simulink model "sf_basic"  (R2015b)
settings: Solver=FixedStepDiscrete  SolverMode=SingleTasking  StartTime=0.0  StopTime=1  RelTol=1e-3
settings Model: Creator=at-mt  LastModifiedBy=amatsumo
settings DataIOCC: SaveFormat=Array  SignalLoggingSaveFormat=ModelDataLogs  SaveOutput=off  SignalLogging=off  SaveTime=off
settings OptimizationCC: BlockReduction=off  ConditionallyExecuteInputs=off  DefaultParameterBehavior=Inlined  ExpressionDepthLimit=2147483647
settings DebuggingCC: AlgebraicLoopMsg=error  UnderspecifiedInitializationDetection=Classic  MergeDetectMultiDrivingBlocksExec=none  SolverPrmCheckMsg=warning  SingleTaskRateTransMsg=error  FcnCallInpInsideContextMsg=UseLocalSettings  StateNameClashWarn=warning
settings HardwareCC: ProdBitPerPointer=32  ProdLargestAtomicFloat=None  ProdIntDivRoundTo=Undefined  ProdEndianess=Unspecified  ProdWordSize=32  ProdHWDeviceType=ASIC/FPGA->ASIC/FPGA  TargetBitPerPointer=64  TargetLongLongMode=on  TargetIntDivRoundTo=Zero  TargetEndianess=LittleEndian  TargetWordSize=64  TargetHWDeviceType=MATLAB Host  ProdEqTarget=off
settings GRTTargetCC: GeneratePreprocessorConditionals=Disable all  CombineOutputUpdateFcns=off  GRTInterface=on
settings ConfigComp: CovModelRefEnable=Off  CovSFcnEnable=off

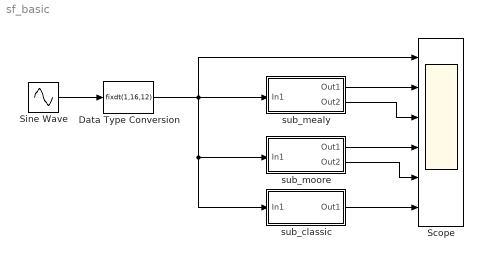
== system sf_basic ==
  Data Type Conversion : DataTypeConversion  OutDataTypeStr=fixdt(1,16,12)
  Scope : Scope  NumInputPorts=6
  Sine Wave : Sin  Amplitude=4  Frequency=20  SampleTime=1/100
  sub_classic : Subsystem
  sub_mealy : Subsystem
  sub_moore : Subsystem
  wires:
  Sine Wave/1 -> Data Type Conversion/1
  sub_mealy/1(Out1) -> Scope/2
  Data Type Conversion/1 -> Scope/1, sub_mealy/1(In1), sub_classic/1(In1), sub_moore/1(In1)
  sub_moore/1(Out1) -> Scope/4
  sub_classic/1(Out1) -> Scope/6
  sub_mealy/2(Out2) -> Scope/3
  sub_moore/2(Out2) -> Scope/5

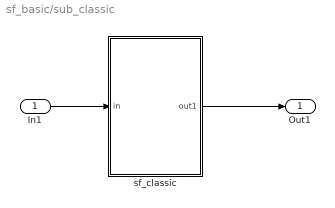
== system sf_basic/sub_classic ==
  In1 : Inport
  sf_classic : Stateflow chart  TreatAsAtomicUnit=on
  Out1 : Outport
  wires:
  In1/1 -> sf_classic/1(in)
  sf_classic/1(out1) -> Out1/1

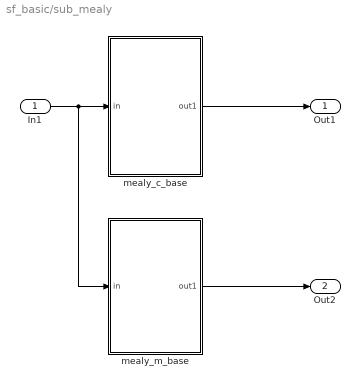
== system sf_basic/sub_mealy ==
  In1 : Inport
  mealy_c_base : Stateflow chart  TreatAsAtomicUnit=on
  mealy_m_base : Stateflow chart  TreatAsAtomicUnit=on
  Out1 : Outport
  Out2 : Outport  Port=2
  wires:
  In1/1 -> mealy_m_base/1(in), mealy_c_base/1(in)
  mealy_c_base/1(out1) -> Out1/1
  mealy_m_base/1(out1) -> Out2/1

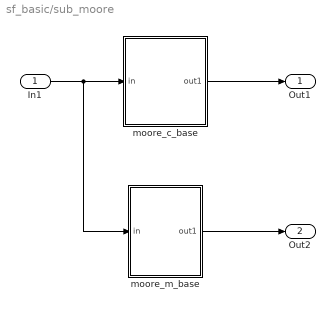
== system sf_basic/sub_moore ==
  In1 : Inport
  moore_c_base : Stateflow chart  TreatAsAtomicUnit=on
  moore_m_base : Stateflow chart  TreatAsAtomicUnit=on
  Out1 : Outport
  Out2 : Outport  Port=2
  wires:
  moore_c_base/1(out1) -> Out1/1
  In1/1 -> moore_m_base/1(in), moore_c_base/1(in)
  moore_m_base/1(out1) -> Out2/1

== stateflow chart sf_basic/sub_mealy/mealy_c_base ==
  settings: updateMethod=DISCRETE  stateMachineType=MEALY_MACHINE  executeAtInitialization=1  initializeOutput=1
  state Init/
  state On1/
  state Off1/
  Init -> Init [order 3] : {out1 = 2;}
  (default) -> Init
  Init -> Off1 [order 2] : [in >= 0]
      | {out1 = 0;}
  On1 -> Init [order 1] : [in >= 0]
      | {out1 = 2;}
  Init -> On1 [order 1] : [in < 0]
      | {out1 = 1;}
  Off1 -> Init [order 1] : [in < 0]
      | {out1 = 2;}
  On1 -> On1 [order 2] : {out1 = 1;}
  Off1 -> Off1 [order 2] : {out1 = 0;}
  data: in input fixdt(1,16,12) size=1; out1 output int16

== stateflow chart sf_basic/sub_moore/moore_m_base ==
  settings: updateMethod=DISCRETE  stateMachineType=MOORE_MACHINE
  state Init/
    out1 = int16(2);
  state On1/
    out1 = int16(1);
  state Off1/
    out1 = int16(0);
  Init -> Init [order 3]
  Init -> Off1 [order 2] : [in >= 0]
  (default) -> Init
  Init -> On1 [order 1] : [in < 0]
  On1 -> Init [order 1] : [in >= 0]
  Off1 -> Init [order 1] : [in < 0]
  On1 -> On1 [order 2]
  Off1 -> Off1 [order 2]
  data: in input fixdt(1,16,12); out1 output int16

== stateflow chart sf_basic/sub_mealy/mealy_m_base ==
  settings: updateMethod=DISCRETE  stateMachineType=MEALY_MACHINE  executeAtInitialization=1  initializeOutput=1
  state Init/
  state On1/
  state Off1/
  Init -> Init [order 3] : {out1 = int16(2);}
  (default) -> Init
  Init -> Off1 [order 2] : [in >= 0]
      | {out1 = int16(0);}
  Init -> On1 [order 1] : [in < 0]
      | {out1 = int16(1);}
  On1 -> Init [order 1] : [in >= 0]
      | {out1 = int16(2);}
  Off1 -> Init [order 1] : [in < 0]
      | {out1 = int16(2);}
  On1 -> On1 [order 2] : {out1 = int16(1);}
  Off1 -> Off1 [order 2] : {out1 = int16(0);}
  data: in input fixdt(1,16,12); out1 output int16

== stateflow chart sf_basic/sub_moore/moore_c_base ==
  settings: updateMethod=DISCRETE  stateMachineType=MOORE_MACHINE  executeAtInitialization=1
  state Init/
    out1 = 2;
  state On1/
    out1 = 1;
  state Off1/
    out1 = 0;
  Init -> Init [order 3]
  Init -> Off1 [order 2] : [in >= 0]
  (default) -> Init
  On1 -> Init [order 1] : [in >= 0]
  Init -> On1 [order 1] : [in < 0]
  Off1 -> Init [order 1] : [in < 0]
  On1 -> On1 [order 2]
  Off1 -> Off1 [order 2]
  data: in input fixdt(1,16,12) size=1; out1 output int16

== stateflow chart sf_basic/sub_classic/sf_classic ==
  settings: updateMethod=DISCRETE  executeAtInitialization=1
  state Init/
    out1 = 2;
  state On1/
    out1 = 1;
  state Off1/
    out1 = 0;
  Init -> Init [order 3]
  Init -> Off1 [order 2] : [in >= 0]
      | {out1 = 0;}
  (default) -> Init
  On1 -> Init [order 1] : [in >= 0]
      | {out1 = 2;}
  Init -> On1 [order 1] : [in < 0]
      | {out1 = 1;}
  Off1 -> Init [order 1] : [in < 0]
      | {out1 = 2;}
  On1 -> On1 [order 2]
  Off1 -> Off1 [order 2]
  data: in input fixdt(1,16,12) size=1; out1 output int16
